simulink model "qpsk"  (R2014a)
settings: Solver=ode45  StartTime=0.0  StopTime=Inf  RelTol=1e-3
libraries: commdigbbndpm3 x2, commfilt2 x2, commseqgen2 x1
settings Model: Creator=ICsomort  LastModifiedBy=ICsomort
settings DebuggingCC: SingleTaskRateTransMsg=error

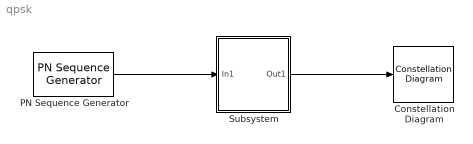
== system qpsk ==
  Constellation Diagram : ConstellationDiagram
  PN Sequence Generator : commseqgen2/PN Sequence Generator  poly=[1 0 0 0 0 1 1]  ini_sta=[0 0 0 0 0 1]  outBitMaskSource=Dialog parameter  shift=0  outVarSiz=off  maxOutSizeMode=Dialog parameter  maxOutSize=[10 1]  Ts=1  frameBased=off  sampPerFrame=1  reset=off  bitPackedOutputs=on  outDataType=double  numPackedBits=2  bitPackDataSigned=off  bitPackedOutDType=Smallest integer
  Subsystem : Subsystem
  wires:
  PN Sequence Generator/1 -> Subsystem/1(In1)
  Subsystem/1(Out1) -> Constellation Diagram/1

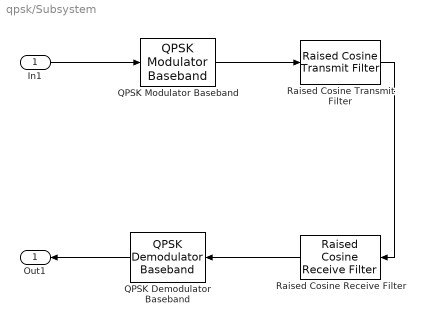
== system qpsk/Subsystem ==
  In1 : Inport  LockScale=on
  QPSK Demodulator Baseband : commdigbbndpm3/QPSK Demodulator Baseband  Ph=pi/4  Dec=Gray  OutType=Integer  DecType=Hard decision  VarSource=Dialog  Variance=1  outDtype1=Inherit via internal rule  outDtype2=Inherit via internal rule  derotateFactorWordLen=16
  QPSK Modulator Baseband : commdigbbndpm3/QPSK Modulator Baseband  InType=Integer  Enc=Gray  Ph=pi/4  outDtype=Fixed-point  outWordLen=16  outUDDataType=sfix(16)  outFracLenMode=Best precision  outFracLen=15
  Raised Cosine Receive Filter : commfilt2/Raised Cosine Receive Filter  filtType=Square root  N=8  filtSpan=6  currentFiltSpan=6  D=(6)/2  R=1  sampMode=Mute  saveAsFlag=0  rateMode=Downsampling  downFactor=8  downOffset=0  framing=Allow multirate processing  InputProcessing=Columns as channels (frame based)  checkGain=Normalized  filterGain=1  checkCoeff=off  launchFVT=on  roundingMode=Floor  overflowMode=off  outputMode=Binary point scaling  outputWordLength=16  outputFracLength=15
  Raised Cosine Transmit Filter : commfilt2/Raised Cosine Transmit Filter  filtType=Square root  filtSpan=6  currentFiltSpan=6  D=(6)/2  R=1  sampMode=Mute  saveAsFlag=0  N=8  framing=Allow multirate processing  InputProcessing=Columns as channels (frame based)  checkGain=Normalized  filterGain=1  checkCoeff=off  launchFVT=on  roundingMode=Floor  overflowMode=off  outputMode=Binary point scaling  outputWordLength=16  outputFracLength=15
  Out1 : Outport
  wires:
  In1/1 -> QPSK Modulator Baseband/1
  QPSK Modulator Baseband/1 -> Raised Cosine Transmit Filter/1
  Raised Cosine Transmit Filter/1 -> Raised Cosine Receive Filter/1
  Raised Cosine Receive Filter/1 -> QPSK Demodulator Baseband/1
  QPSK Demodulator Baseband/1 -> Out1/1
